simulink model "slexFMCWMultiTargetsDOAExample"  (R2018b)
settings: Solver=FixedStepDiscrete  StartTime=0.0  StopTime=512*paramFMCWRSA.T  RelTol=1e-3  EnableMultiTasking=on
PreLoadFcn:
  | helperslexFMCWMultiTargetsDOAParam
undefined symbols (not defined in the file or in its folder): paramFMCWRSA, phased
libraries: phasedenvlib x5, phasedtxrxlib x4, dspsigattribs x2, phasedwavlib x1, phaseddetectlib x1, phasedbflib x1
CloseFcn:
  | clear paramFMCWRSA
settings Model: Creator=The MathWorks, Inc.  LastModifiedBy=The MathWorks, Inc.
settings DataIOCC: LimitDataPoints=on  SaveFormat=StructureWithTime
settings OptimizationCC: LifeSpan=inf
settings DebuggingCC: SFUnexpectedBacktrackingDiag=warning  SFNoUnconditionalDefaultTransitionDiag=warning  SFExecutionAtInitializationDiag=none
settings HardwareCC: ProdBitPerPointer=32  ProdBitPerSizeT=32  ProdBitPerPtrDiffT=32  ProdLargestAtomicFloat=None  ProdIntDivRoundTo=Undefined  ProdEndianess=Unspecified  ProdWordSize=32  ProdHWDeviceType=32-bit Generic
settings ModelReferenceCC: PropagateSignalLabelsOutOfModel=off
settings SFSimCC: SimUseLocalCustomCode=off
settings RTWCC: RTWUseLocalCustomCode=off
settings CodeAppCC: StateflowObjectComments=on
settings GRTTargetCC: TargetLangStandard=C89/C90 (ANSI)  GeneratePreprocessorConditionals=Disable all
settings ConfigComp: CovMetricSettings=dw  CovHtmlReporting=on  CovSaveCumulativeToWorkspaceVar=on  CovSaveSingleToWorkspaceVar=on  CovExternalEMLEnable=off

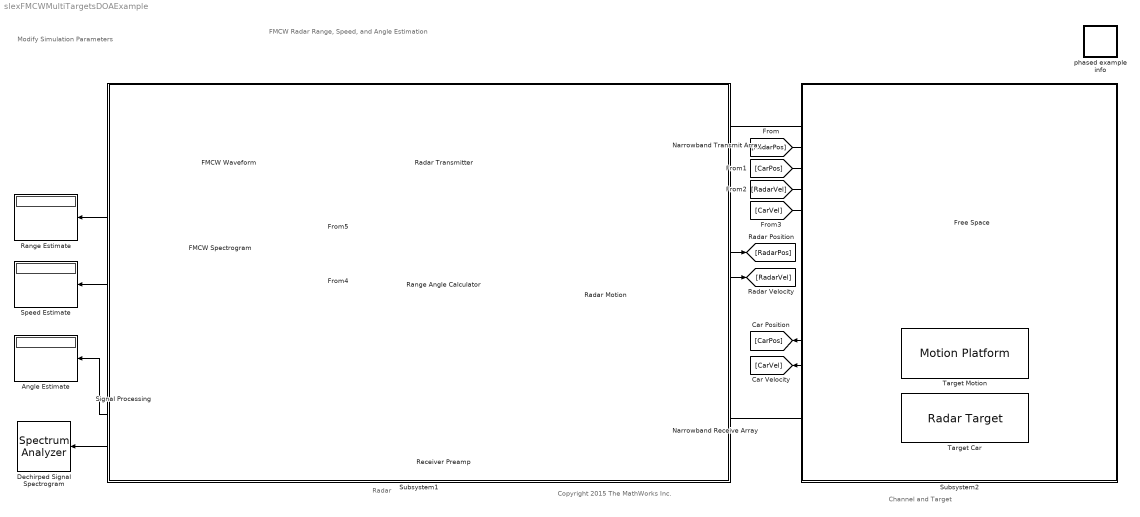
== system slexFMCWMultiTargetsDOAExample ==
  note: Radar
  note: Channel and Target
  note: FMCW Radar Range, Speed, and Angle Estimation
  note: Modify Simulation Parameters
  note: Copyright 2015 The MathWorks Inc.
  Angle Estimate : Display
  Dechirped Signal Spectrogram : SpectrumAnalyzer
  FMCW Spectrogram : SpectrumAnalyzer
  FMCW Waveform : phasedwavlib/FMCW Waveform  SampleRate=paramFMCWRSA.Fs  SweepTime=paramFMCWRSA.T  SweepBandwidth=paramFMCWRSA.Fs  SweepDirection=Up  SweepInterval=Symmetric  OutputFormat=Sweeps  NumSamples=100  NumSweeps=1  SimulateUsing=Interpreted execution
      settings: SourceProductName=Phased Array System Toolbox  SourceProductBaseCode=AR
  Free Space : phasedenvlib/Free Space  PropagationSpeed=paramFMCWRSA.C  OperatingFrequency=paramFMCWRSA.Fc  TwoWayPropagation=on  SampleRateFromInputCheckbox=on  SampleRate=1e6  MaximumDistanceSource=Property  MaximumDistance=10e3  MaximumNumInputSamplesSource=Auto  MaximumNumInputSamples=1000  SimulateUsing=Interpreted execution
      settings: SourceProductName=Phased Array System Toolbox  SourceProductBaseCode=AR
  Narrowband Receive Array : phasedtxrxlib/Narrowband Receive Array  PropagationSpeed=paramFMCWRSA.C  OperatingFrequency=paramFMCWRSA.Fc  Wavefront=Plane  SensorGainMeasure=dB  Polarization=None  WeightsInputPort=off  SimulateUsing=Interpreted execution  Sensor=phased.ULA('Element',phased.IsotropicAntennaElement(),'NumElements',4,'ElementSpacing',0.5*paramFMCWRSA.lambda)
      settings: SourceProductName=Phased Array System Toolbox  SourceProductBaseCode=AR
  Narrowband Transmit Array : phasedtxrxlib/Narrowband Transmit Array  PropagationSpeed=paramFMCWRSA.C  OperatingFrequency=paramFMCWRSA.Fc  CombineRadiatedSignals=on  SensorGainMeasure=dB  Polarization=None  WeightsInputPort=off  SimulateUsing=Interpreted execution  Sensor=phased.ULA('Element',phased.IsotropicAntennaElement(),'NumElements',4,'ElementSpacing',0.5*paramFMCWRSA.lambda)
      settings: SourceProductName=Phased Array System Toolbox  SourceProductBaseCode=AR
  Radar Motion : phasedenvlib/Motion Platform  MotionModel=Velocity  InitialPosition=paramFMCWRSA.RadarPos  InitialVelocity=[ 0; 0; 0 ]  VelocitySource=Property  Velocity=paramFMCWRSA.RadarVel  AccelerationSource=Property  Acceleration=[0;0;0]  CustomTrajectory=[ 0, 0, 0, 0, 0, 0, 0; 1, 0, 0, 0, 0, 0, 0 ]  ScanMode=None  InitialScanAngle=0  AzimuthSpan=[ -60, 60 ]  AzimuthScanRate=10  InitialOrientationAxes=eye( 3 )  OrientationAxesOutputPort=off  ElapsedTimeSource=Auto  SampleRateFromInputCheckbox=on  SampleRate=1e6  SimulateUsing=Interpreted execution
      settings: SourceProductName=Phased Array System Toolbox  SourceProductBaseCode=AR
  Radar Transmitter : phasedtxrxlib/Transmitter  PeakPower=paramFMCWRSA.ppow  Gain=paramFMCWRSA.TxGain  LossFactor=0  InUseOutputPort=off  CoherentOnTransmit=on  PhaseNoiseOutputPort=off  SeedSource=Auto  Seed=0  SimulateUsing=Interpreted execution
      settings: SourceProductName=Phased Array System Toolbox  SourceProductBaseCode=AR
  Range Angle Calculator : phasedenvlib/Range Angle Calculator  Model=Free space  ReferencePositionSource=Input port  ReferencePosition=[ 0; 0; 0 ]  ReferenceAxesSource=Property  ReferenceAxes=eye( 3 )  Output=Angle  SimulateUsing=Interpreted execution
      settings: SourceProductName=Phased Array System Toolbox  SourceProductBaseCode=AR
  Range Estimate : Display
  Receiver Preamp : phasedtxrxlib/Receiver Preamp  Gain=paramFMCWRSA.RxGain  LossFactor=0  NoiseMethod=Noise temperature  NoiseFigure=paramFMCWRSA.NF  ReferenceTemperature=290  SampleRateFromInputCheckbox=on  SampleRate=1e6  NoisePower=0  EnableInputPort=off  PhaseNoiseInputPort=off  SeedSource=Auto  Seed=0  SimulateUsing=Interpreted execution
      settings: SourceProductName=Phased Array System Toolbox  SourceProductBaseCode=AR
  Signal Processing : Subsystem
      mask Display:
      | disp('Signal\nProcessing')
      | port_label('input',1,'Ref')
      | port_label('input',2,'Echo')
      | port_label('output',1,'Rng')
      | port_label('output',2,'Vel')
      | port_label('output',4,'Dechirped')
      | port_label('output',3,'Ang')
  Speed Estimate : Display
  Subsystem1 : Subsystem
  Subsystem2 : Subsystem
  Target Car : phasedenvlib/Radar Target  EnablePolarization=off  Mode=Monostatic  MeanRCSSource=Property  ScatteringMatrixSource=Property  MeanRCS=paramFMCWRSA.RCS  ScatteringMatrix=eye( 2 )  Model=Nonfluctuating  PropagationSpeed=paramFMCWRSA.C  OperatingFrequency=paramFMCWRSA.Fc  SeedSource=Auto  Seed=0  SimulateUsing=Interpreted execution
      settings: SourceProductName=Phased Array System Toolbox  SourceProductBaseCode=AR
  Target Motion : phasedenvlib/Motion Platform  MotionModel=Velocity  InitialPosition=paramFMCWRSA.CarPos  InitialVelocity=[ 0; 0; 0 ]  VelocitySource=Property  Velocity=paramFMCWRSA.CarVel  AccelerationSource=Property  Acceleration=[0;0;0]  CustomTrajectory=[ 0, 0, 0, 0, 0, 0, 0; 1, 0, 0, 0, 0, 0, 0 ]  ScanMode=None  InitialScanAngle=0  AzimuthSpan=[ -60, 60 ]  AzimuthScanRate=10  InitialOrientationAxes=eye( 3 )  OrientationAxesOutputPort=off  ElapsedTimeSource=Auto  SampleRateFromInputCheckbox=on  SampleRate=1e6  SimulateUsing=Interpreted execution
      settings: SourceProductName=Phased Array System Toolbox  SourceProductBaseCode=AR
  phased example info : Subsystem
      settings: OpenFcn=|
      | modelname = 'slexFMCWExample';
      | helpview(fullfile(matlabroot,'help','phased','helptargets.map'),sprintf('%sExample',modelname));
      | clear modelname;
      mask Display: disp('Info')
  wires:
  FMCW Waveform/1 -> Radar Transmitter/1, Signal Processing/1(In1), FMCW Spectrogram/1
  [RadarPos] -> Free Space/2
  [CarPos] -> Free Space/3
  [RadarVel] -> Free Space/4
  [CarVel] -> Free Space/5
  Radar Motion/1 -> [RadarPos]
  Radar Motion/2 -> [RadarVel]
  Free Space/1 -> Target Car/1
  Target Motion/1 -> [CarPos]
  Target Motion/2 -> [CarVel]
  Receiver Preamp/1 -> Signal Processing/2(In2)
  Radar Transmitter/1 -> Narrowband Transmit Array/1
  Narrowband Transmit Array/1 -> Free Space/1
  Narrowband Receive Array/1 -> Receiver Preamp/1
  Target Car/1 -> Narrowband Receive Array/1
  [CarPos] -> Range Angle Calculator/1
  [RadarPos] -> Range Angle Calculator/2
  Range Angle Calculator/1 -> Narrowband Receive Array/2, Narrowband Transmit Array/2
  Signal Processing/4(Out4) -> Dechirped Signal Spectrogram/1
  Signal Processing/3(Out3) -> Angle Estimate/1
  Signal Processing/2(Out2) -> Speed Estimate/1
  Signal Processing/1(Out1) -> Range Estimate/1

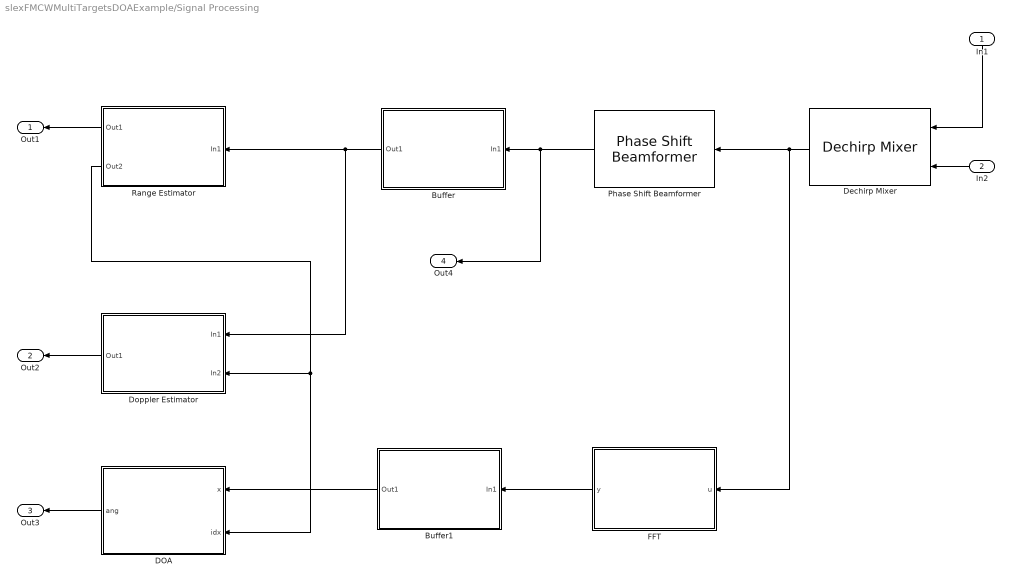
== system slexFMCWMultiTargetsDOAExample/Signal Processing ==
  In1 : Inport
  In2 : Inport  Port=2
  Buffer : Subsystem
  Buffer1 : Subsystem
  DOA : MATLAB Function  TreatAsAtomicUnit=on  mask(DOA Estimation){Ne=4, Ns=2048, c=paramFMCWRSA.C, fc=paramFMCWRSA.Fc}
      mask prompts: Ne "Number of Antennas"; Ns "Number of FFT Points in Range"; c "Propagation Speed (m/s)"; fc "Operating Frequency (Hz)"
      mask help: Estimate the target direction
  Dechirp Mixer : phaseddetectlib/Dechirp Mixer
      settings: SourceProductName=Phased Array System Toolbox  SourceProductBaseCode=AR
  Doppler Estimator : Subsystem  mask(Doppler Estimation){N=2048, lambda=paramFMCWRSA.lambda}
      mask prompts: N "Number of FFT Points"; lambda "Wavelength (m)"
      mask help: Estiamte the target speed
      mask Display:
      | disp('Doppler\n Estimator')
      | port_label('input',1,'X')
      | port_label('input',2,'Idx')
      | port_label('output',1,'Vel')
  FFT : MATLAB Function  TreatAsAtomicUnit=on  mask{N=2048}
      mask prompts: N "Number of FFT Points"
  Phase Shift Beamformer : phasedbflib/Phase Shift Beamformer  PropagationSpeed=paramFMCWRSA.C  OperatingFrequency=paramFMCWRSA.Fc  DirectionSource=Property  Direction=[ 0; 0 ]  NumPhaseShifterBits=0  WeightsNormalization=Distortionless  WeightsOutputPort=off  SimulateUsing=Interpreted execution  SensorArray=phased.ULA('Element',phased.IsotropicAntennaElement(),'NumElements',4,'ElementSpacing',0.5*paramFMCWRSA.lambda)
      settings: SourceProductName=Phased Array System Toolbox  SourceProductBaseCode=AR
  Range Estimator : Subsystem  mask(Range Estimator){c=paramFMCWRSA.C, k=paramFMCWRSA.Fs/paramFMCWRSA.T, N=2048}
      mask prompts: c "Propagation Speed (m/s)"; k "FMCW Sweep Slope (Hz/s)"; N "Number of FFT Points"
      mask help: Compute periodogram of the incoming signal, find the beat frequency, and convert the beat frequency to the range estimate.
      mask Display:
      | disp('Range\nEstimator')
      | port_label('input',1,'X')
      | port_label('output',1,'Rng')
      | port_label('output',2,'Idx')
  Out1 : Outport
  Out2 : Outport  Port=2
  Out3 : Outport  Port=3
  Out4 : Outport  Port=4
  wires:
  In1/1 -> Dechirp Mixer/1
  In2/1 -> Dechirp Mixer/2
  Range Estimator/1(Out1) -> Out1/1
  Dechirp Mixer/1 -> FFT/1(u), Phase Shift Beamformer/1
  Doppler Estimator/1(Out1) -> Out2/1
  Buffer/1(Out1) -> Doppler Estimator/1(In1), Range Estimator/1(In1)
  Range Estimator/2(Out2) -> DOA/2(idx), Doppler Estimator/2(In2)
  Phase Shift Beamformer/1 -> Out4/1, Buffer/1(In1)
  FFT/1(y) -> Buffer1/1(In1)
  Buffer1/1(Out1) -> DOA/1(x)
  DOA/1(ang) -> Out3/1

== system slexFMCWMultiTargetsDOAExample/Subsystem1 ==

== system slexFMCWMultiTargetsDOAExample/Subsystem2 ==

== system slexFMCWMultiTargetsDOAExample/phased example info ==

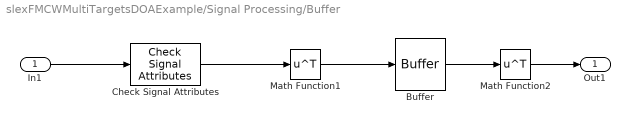
== system slexFMCWMultiTargetsDOAExample/Signal Processing/Buffer ==
  In1 : Inport
  Buffer : Buffer
  Check Signal Attributes : dspsigattribs/Check Signal Attributes  SigAttribCheckMethod=Does not match attributes exactly  Complexity=Ignore  Frame=Ignore  DimsCheckMethod=Is...  Dimensions=Column vector (2-D) or scalar  DatatypeCheckMethod=Ignore  DatatypeGeneral=Boolean  DtypeFloatSpecific=Any floating-point  DtypeFixedSpecific=Any fixed-point  DtypeIntSpecific=Any integer  SampleMode=Ignore
      settings: SourceProductName=DSP System Toolbox  SourceProductBaseCode=DS
  Math Function1 : Math  Operator=transpose  OutputSignalType=complex  SaturateOnIntegerOverflow=on
  Math Function2 : Math  Operator=transpose  OutputSignalType=complex  SaturateOnIntegerOverflow=on
  Out1 : Outport
  wires:
  Check Signal Attributes/1 -> Math Function1/1
  Math Function2/1 -> Out1/1
  Math Function1/1 -> Buffer/1
  In1/1 -> Check Signal Attributes/1
  Buffer/1 -> Math Function2/1

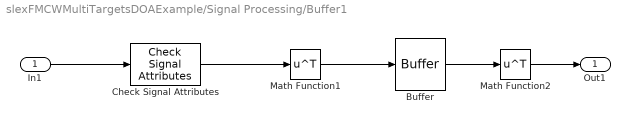
== system slexFMCWMultiTargetsDOAExample/Signal Processing/Buffer1 ==
  In1 : Inport
  Buffer : Buffer
  Check Signal Attributes : dspsigattribs/Check Signal Attributes  SigAttribCheckMethod=Does not match attributes exactly  Complexity=Ignore  Frame=Ignore  DimsCheckMethod=Is...  Dimensions=Column vector (2-D) or scalar  DatatypeCheckMethod=Ignore  DatatypeGeneral=Boolean  DtypeFloatSpecific=Any floating-point  DtypeFixedSpecific=Any fixed-point  DtypeIntSpecific=Any integer  SampleMode=Ignore
      settings: SourceProductName=DSP System Toolbox  SourceProductBaseCode=DS
  Math Function1 : Math  Operator=transpose  OutputSignalType=complex  SaturateOnIntegerOverflow=on
  Math Function2 : Math  Operator=transpose  OutputSignalType=complex  SaturateOnIntegerOverflow=on
  Out1 : Outport
  wires:
  Buffer/1 -> Math Function2/1
  In1/1 -> Check Signal Attributes/1
  Math Function1/1 -> Buffer/1
  Math Function2/1 -> Out1/1
  Check Signal Attributes/1 -> Math Function1/1

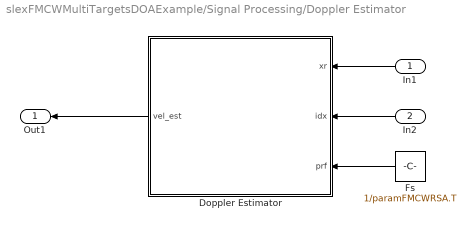
== system slexFMCWMultiTargetsDOAExample/Signal Processing/Doppler Estimator ==
  In1 : Inport
  In2 : Inport  Port=2
  Doppler Estimator : MATLAB Function  TreatAsAtomicUnit=on
  Fs : Constant  Value=1/paramFMCWRSA.T
  Out1 : Outport
  wires:
  Doppler Estimator/1(vel_est) -> Out1/1
  Fs/1 -> Doppler Estimator/3(prf)
  In1/1 -> Doppler Estimator/1(xr)
  In2/1 -> Doppler Estimator/2(idx)

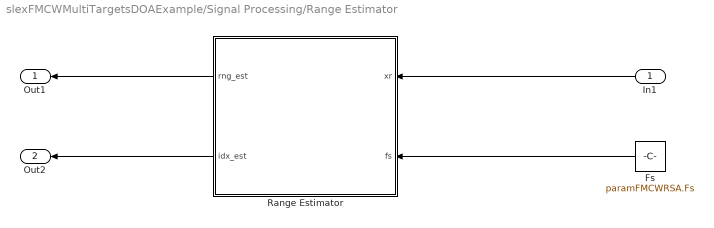
== system slexFMCWMultiTargetsDOAExample/Signal Processing/Range Estimator ==
  In1 : Inport
  Fs : Constant  Value=paramFMCWRSA.Fs
  Range Estimator : MATLAB Function  TreatAsAtomicUnit=on
  Out1 : Outport
  Out2 : Outport  Port=2
  wires:
  Range Estimator/1(rng_est) -> Out1/1
  In1/1 -> Range Estimator/1(xr)
  Fs/1 -> Range Estimator/2(fs)
  Range Estimator/2(idx_est) -> Out2/1

== matlab function slexFMCWMultiTargetsDOAExample/Signal Processing/Doppler Estimator/Doppler Estimator ==
  data: xr input; idx input; prf input; N parameter; lambda parameter; vel_est output
function vel_est = fcn(xr,idx,prf,N,lambda)
%#codegen

vel_est = zeros(3,1);
if idx(1)~=1
    rngdata = fftshift(fft(xr,N,1),1);
    fdop = prf*(-0.5+(0:N-1)/N);
    for m = 1:3
        dopdata = fftshift(fft(rngdata(idx(m),:),N,2),2);
        Pd = abs(dopdata);
        [~,dopidx] = findpeaks(Pd,'NPeaks',1,'SortStr','descend');
        vel_est(m) = fdop(dopidx(1));
    end
    vel_est = -dop2speed(vel_est,lambda)/2;
end

== matlab function slexFMCWMultiTargetsDOAExample/Signal Processing/DOA ==
  data: x input; ang output; idx input; Ne parameter; Ns parameter; c parameter; fc parameter
function ang = fcn(x,idx,Ne,Ns,c,fc)
%#codegen

persistent doa;
if isempty(doa)
    doa = phased.RootMUSICEstimator(...
        'SensorArray',phased.ULA(4,0.5*c/fc),...
        'OperatingFrequency',fc,'PropagationSpeed',c,...
        'NumSignalsSource','Property','NumSignals',1);
end
ang = zeros(3,1);
if idx(1)~=1
    for m = 1:3
        ang(m) = step(doa,x(idx(m)+(0:Ne-1)*Ns,:)');  % conj due to the order of dechirp
    end
end

== matlab function slexFMCWMultiTargetsDOAExample/Signal Processing/FFT ==
  data: u input; y output; N parameter
function y = fcn(u,N)
%#codegen

yf = fftshift(fft(u,N,1),1);
y = yf(:);

== matlab function slexFMCWMultiTargetsDOAExample/Signal Processing/Range Estimator/Range Estimator ==
  data: xr input; rng_est output; fs input; k parameter; c parameter; N parameter; idx_est output
function [rng_est,idx_est] = fcn(xr,fs,k,c,N)
%#codegen

f = fs*(-0.5+(0:N-1)/N);
rngdata = fftshift(fft(xr,N,1),1);
P = abs(sum(rngdata,2));
[~,idx] = findpeaks(P,'NPeaks',3,'SortStr','descend','MinPeakDistance',10);
if numel(idx) == 3
    fb_rng = f(idx(1:3));
    rng_est = beat2range(fb_rng(:),k,c);
    idx_est = zeros(3,1);
    idx_est(1:3) = idx(1:3);
   
else
    rng_est = [0; 0; 0];
    idx_est = [1; 1; 1];
end
